simulink model "closedloop_model_ClampingWindup"  (R2024a)
settings: Solver=ode45  StartTime=0.0  StopTime=10  RelTol=1e-4  AbsTol=1e-4
undefined symbols (not defined in the file): F_den, F_num, G_den, G_num, Kp, Td, Ti
settings Model: SimulationMode=accelerator  Creator=thoma  LastModifiedBy=thoma

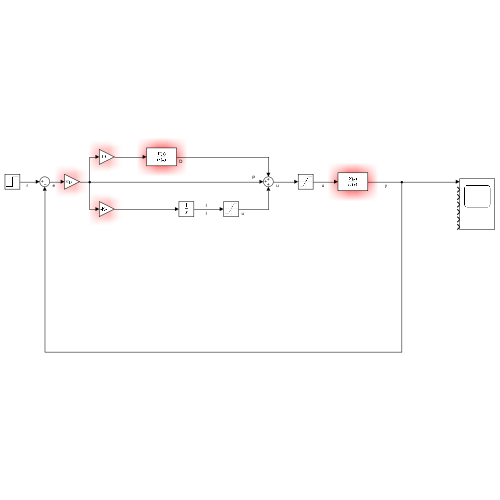
[thumbnail: Simulink's stored preview of the top-level diagram]
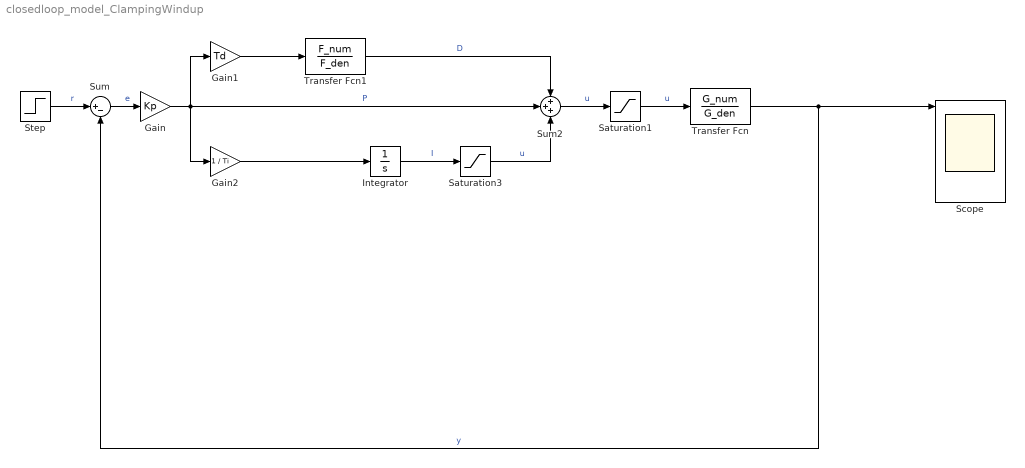
== system closedloop_model_ClampingWindup ==
  Gain : Gain  Gain=Kp
  Gain1 : Gain  Gain=Td
  Gain2 : Gain  Gain=1 / Ti
  Integrator : Integrator
  Saturation1 : Saturate  UpperLimit=5  LowerLimit=-5
  Saturation3 : Saturate  UpperLimit=5  LowerLimit=-5
  Scope : Scope  NumInputPorts=7
  Step : Step  Time=0  SampleTime=0
  Sum : Sum  Inputs=|+-
  Sum2 : Sum  Inputs=+++
  Transfer Fcn : TransferFcn  Numerator=G_num  Denominator=G_den
  Transfer Fcn1 : TransferFcn  Numerator=F_num  Denominator=F_den
  wires:
  Gain/1 -> Sum2/2, Gain1/1, Gain2/1  "P"
  Step/1 -> Sum/1  "r"
  Gain1/1 -> Transfer Fcn1/1
  Transfer Fcn1/1 -> Sum2/1  "D"
  Transfer Fcn/1 -> Sum/2, Scope/1  "y"
  Sum2/1 -> Saturation1/1  "u"
  Saturation1/1 -> Transfer Fcn/1  "u"
  Integrator/1 -> Saturation3/1  "I"
  Sum/1 -> Gain/1  "e"
  Gain2/1 -> Integrator/1
  Saturation3/1 -> Sum2/3  "u"
